simulink model "top_model"  (R2018a)
settings: Solver=VariableStepAuto  StartTime=0.0  StopTime=10.0  RelTol=1e-3  EnableMultiTasking=on
undefined symbols (not defined in the file): m, n
settings Model: Creator=The MathWorks, Inc.  LastModifiedBy=rl185160
settings DataIOCC: LimitDataPoints=on
settings OptimizationCC: LifeSpan=inf
settings DebuggingCC: AllowSymbolicDim=off  SFUnexpectedBacktrackingDiag=warning  SFNoUnconditionalDefaultTransitionDiag=warning  SFExecutionAtInitializationDiag=none
settings ModelReferenceCC: PropagateSignalLabelsOutOfModel=off
settings CodeAppCC: StateflowObjectComments=on
settings GRTTargetCC: TargetLangStandard=C89/C90 (ANSI)
settings ConfigComp: CovMetricSettings=dw  CovHtmlReporting=on  CovSaveCumulativeToWorkspaceVar=on  CovSaveSingleToWorkspaceVar=on  CovExternalEMLEnable=off

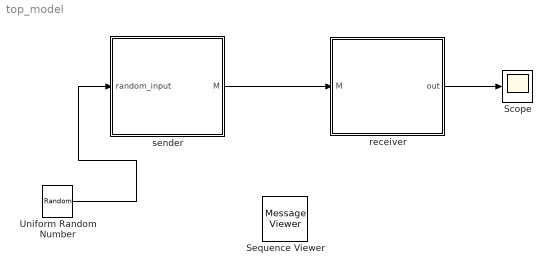
== system top_model ==
  Scope : Scope
  Sequence Viewer : MessageViewer
  Uniform Random Number : UniformRandomNumber  Seed=0.1  SampleTime=0.1
  receiver : Stateflow chart  TreatAsAtomicUnit=on
  sender : Stateflow chart  TreatAsAtomicUnit=on
  wires:
  receiver/1(out) -> Scope/1
  sender/1(M) -> receiver/1(M)
  Uniform Random Number/1 -> sender/1(random_input)

== stateflow chart top_model/receiver ==
  state Ready
  state Processing
    entry:
    % do computation
    if M.data > 0
    out = 1
    else
    out = -1
    end
  (default) -> Ready
  Processing -> Ready : [after(0.1,sec)]
  Ready -> Processing : M % check message in the queue
  data: out output; M input

== stateflow chart top_model/sender ==
  state Wait
  state Produce
    entry: x = x + 0.2;
    M.data = sin(x);
  state Send
    entry:
    send(M);
  (default) -> Wait
  Wait -> Produce : [random_input > 0]{ x = 1;}
      | % creates random interval
  Send -> Wait
  Produce -> Send
  data: random_input input; x local; M output
